simulink model "RobotMovil_SCST"  (R2021a)
settings: Solver=VariableStepAuto  StartTime=0.0  StopTime=25  RelTol=1e-3
model workspace: external: MATLAB File G:\My Drive\0. PUCP\Cursos\2020.2\IEE243 - Sistemas de Control\Tarea Academica\Simulacion Robot Movil\cad files\RobotMovil_DataFile.m (data not in the file)
undefined symbols (not defined in the file): smiData, X, xPla, Y, yPla, Z, zPla
libraries: sm_lib x211, nesl_utility x6, simulink x3, fl_lib x3
(part 5 of 5)

== system RobotMovil_SCST/MODELO CINEMÁTICO ROBOT MOVIL/RobotMovilBase_2_RIGID/shield_rb_1_RIGID/shield_rb_step_1_RIGID/tc_3528_step_1_RIGID ==
  ReferenceFrame : sm_lib/Frames and Transforms/Reference Frame
  Solid : sm_lib/Body Elements/File Solid  ExtGeomFileName=tc_3528.step_Default_sldprt.STEP  UnitType=FromFile  ExtGeomFileUnits=m  StepReaderType=HEX  ExportConvexHullGeometry=off  InertiaType=Custom  Mass=smiData.Solid(7).mass  MassUnits=kg  CenterOfMass=smiData.Solid(7).CoM  CenterOfMassUnits=mm  MomentsOfInertia=smiData.Solid(7).MoI  MomentsOfInertiaUnits=kg*mm^2  ProductsOfInertia=smiData.Solid(7).PoI  ProductsOfInertiaUnits=kg*mm^2  BasedOnType=DensityFromFile  Density=1000  DensityUnits=kg/m^3  DoExposeReferenceFrame=on  SerializedFrames=<Frames/>  GraphicType=FromGeometry  MarkerShape=Sphere  MarkerSize=10  GraphicVisPropType=SimpleVisualProperties  GraphicDiffuseColor=smiData.Solid(7).color  GraphicSpecularColor=[0.5 0.5 0.5 1.0]  GraphicAmbientColor=[0.15 0.15 0.15 1.0]  GraphicEmissiveColor=[0.0 0.0 0.0 1.0]  GraphicShininess=75  GraphicOpacity=smiData.Solid(7).opacity
  F : PMIOPort  Side=Left
  connections:
  Solid/RConn1 -- ReferenceFrame/RConn1 -- F/RConn1

== matlab function RobotMovil_SCST/Conversion ==
  data: w_ref input; u_ref input; wd_ref output; wi_ref output
function [wd_ref, wi_ref] = fcn(w_ref, u_ref)
r=0.0345;
d=0.147;
%a=d/2;

wd_ref = (2*u_ref+d*w_ref)/(2*r);
wi_ref = 2*u_ref/r-wd_ref;

== matlab function RobotMovil_SCST/Sistema de Control de Velocidad ==
  data: wd input; wi input; wd_ref input; ud output; wi_ref input; ui output
function [ud, ui] = fcn(wd,wi,wd_ref,wi_ref)
persistent ud_1
persistent ed_1
persistent ui_1
persistent ei_1
if isempty(ud_1)
    ud_1=0;
    ed_1=0;
    ui_1=0;
    ei_1=0;
end
%Motor Derecha (Claudia)
%Cuidado que  wd_ref, wi_ref pueden estar en radianes
ed=wd_ref-wd;
Ts_d=0.01;
Kp_d = 0.0208;
Ki_d = 0.1248;
ud=ud_1+(2*Kp_d+Ki_d*Ts_d)/2*ed+(Ki_d*Ts_d-2*Kp_d)/2*ed_1;
ed_1=ed;
ud_1=ud;

%Motor Izquierda (Pierre)
%Cuidado que  wd_ref, wi_ref pueden estar en radianes
ei=wi_ref-wi;
Ts_i=0.006;
Kp_i=0.020056241439231;
Ki_i=0.441237311663075;
ui=ui_1+(2*Kp_i+Ki_i*Ts_i)/2*ei+(Ki_i*Ts_i-2*Kp_i)/2*ei_1;
ei_1=ei;
ui_1=ui;

== matlab function RobotMovil_SCST/Controlador de Seguimiento de Trayectoria ==
  data: xd input; yd input; xdp input; w_ref output; ydp input; x input; y input; u_ref output; phi input
function [w_ref, u_ref] = fcn(xd,yd,xdp,ydp,x,y,phi)

a = 0.147/2;
K1 = 1;%Tes=4 seg
K2 = 1;%Tes=4 seg
%phi en radianes
xa = x + a*cos(phi);
ya = y + a*sin(phi);
%definimos la matriz M
detM=a;
Minv_11 = a*cos(phi)/detM;
Minv_12 = a*sin(phi)/detM;
Minv_21 = -sin(phi)/detM;
Minv_22 = cos(phi)/detM;
%
av1 = xdp + K1*(xd-xa);
av2 = ydp + K2*(yd-ya);
%
u_ref = Minv_11*av1 + Minv_12*av2;
w_ref = Minv_21*av1 + Minv_22*av2;%está radianes

== matlab function RobotMovil_SCST/Trayectoria ==
  data: u input; xd output; yd output; xdp output; ydp output
function [xd,yd,xdp,ydp] = fcn(u)

persistent t

if isempty(t)
    t=0;
end
R=20;
xd =R*cos(t);
yd =R*sin(t);

xdp =0.1;
ydp =0.1;

t = t + 0.07;

== matlab function RobotMovil_SCST/MATLAB Function ==
  data: x input; xa output; y input; phi input; ya output
function [xa,ya] = fcn(x,y,phi)

a = 0.147/2;

xa = x + a*cos(phi);
ya = y + a*sin(phi);
